simulink model "simu_contr_digit"  (R2021a)
settings: Solver=VariableStepAuto  StartTime=0.0  StopTime=3  RelTol=1e-3
libraries: cstblocks x6
settings Model: Creator=frand  LastModifiedBy=frand

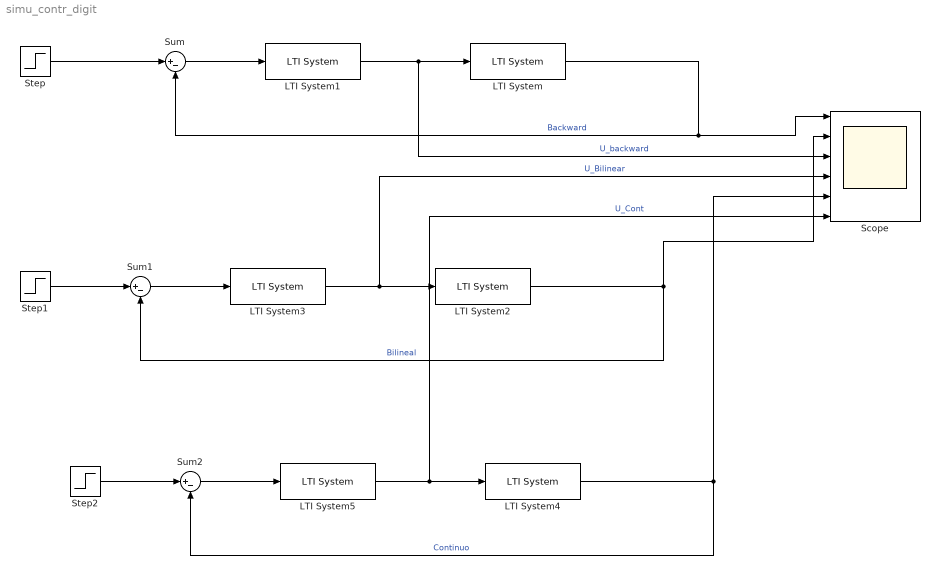
== system simu_contr_digit ==
  LTI System : cstblocks/LTI System  sys=P  IC=[]
  LTI System1 : cstblocks/LTI System  sys=C_back  IC=[]
  LTI System2 : cstblocks/LTI System  sys=P  IC=[]
  LTI System3 : cstblocks/LTI System  sys=C_bil  IC=[]
  LTI System4 : cstblocks/LTI System  sys=P  IC=[]
  LTI System5 : cstblocks/LTI System  sys=C  IC=[]
  Scope : Scope  NumInputPorts=6
  Step : Step  SampleTime=0
  Step1 : Step  SampleTime=0
  Step2 : Step  SampleTime=0
  Sum : Sum  Inputs=|+-
  Sum1 : Sum  Inputs=|+-
  Sum2 : Sum  Inputs=|+-
  wires:
  Step/1 -> Sum/1
  Sum/1 -> LTI System1/1
  LTI System1/1 -> Scope/3, LTI System/1  "U_backward"
  LTI System/1 -> Sum/2, Scope/1  "Backward"
  LTI System2/1 -> Scope/2, Sum1/2  "Bilineal"
  LTI System3/1 -> Scope/4, LTI System2/1  "U_Bilinear"
  Sum1/1 -> LTI System3/1
  Step1/1 -> Sum1/1
  Step2/1 -> Sum2/1
  Sum2/1 -> LTI System5/1
  LTI System5/1 -> Scope/6, LTI System4/1  "U_Cont"
  LTI System4/1 -> Scope/5, Sum2/2  "Continuo"
